simulink model "progetto_condizionatore_pid"  (R2022a)
settings: Solver=VariableStepAuto  StartTime=0.0  StopTime=50000  RelTol=1e-3
values from neighbouring files (symbols this model uses):
  A = [(-gamma_cs/C_c) (gamma_cs/C_c); (gamma_cs/C_s) -((gamma_cs/C_s)+(gamma_sa/C_s))]    [Progetto_condizionatore.m]
  B = [1/C_c; 0]    [Progetto_condizionatore.m]
  C = [0 1]    [Progetto_condizionatore.m]
  C_s = 45225    [Progetto_condizionatore.m]
  D = 0    [Progetto_condizionatore.m]
  gamma_sa = 2.3    [Progetto_condizionatore.m]
  temp_amb = 30    [Progetto_condizionatore.m]
libraries: slpidlib x1
settings Model: Creator=Mattia  LastModifiedBy=Mattia

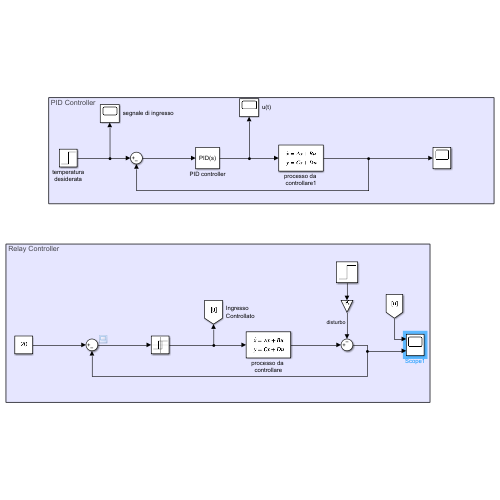
[thumbnail: Simulink's stored preview of the top-level diagram]
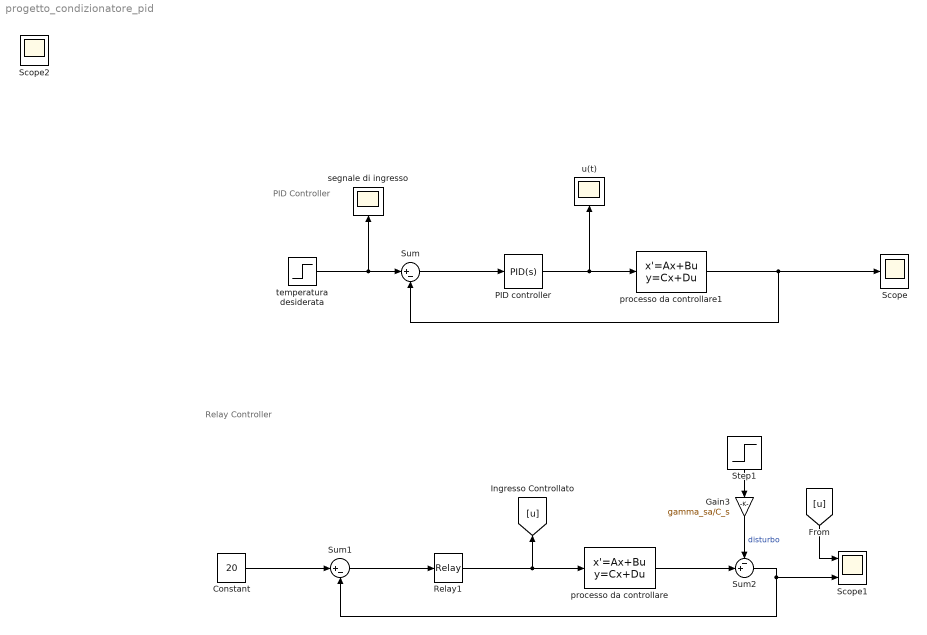
== system progetto_condizionatore_pid ==
  note: Relay Controller
  note: PID Controller
  Constant : Constant  Value=20
  Gain3 : Gain  Gain=gamma_sa/C_s
  PID controller : slpidlib/PID Controller  Controller=PID  Form=Parallel  TimeDomain=Continuous-time  UseExternalTs=off  SampleTime=-1  IntegratorMethod=Forward Euler  FilterMethod=Forward Euler  ControllerParametersSource=internal  P=18  I=0.01  UseKiTs=off  D=0.1  N=100  UseFilter=on  TunerSelectOption=Transfer Function Based (PID Tuner App)  InitialConditionSource=internal  InitialConditionForIntegrator=0  InitialConditionForFilter=0  DifferentiatorICPrevScaledInput=0  ExternalReset=none  TrackingMode=off  Kt=1  LimitOutput=off  SatLimitsSource=internal  UpperSaturationLimit=inf  LowerSaturationLimit=-inf  LinearizeAsGain=on  AntiWindupMode=none  Kb=1  POutMin=[]  POutMax=[]  IOutMin=[]  IOutMax=[]  DOutMin=[]  DOutMax=[]  NOutMin=[]  NOutMax=[]  SumOutMin=[]  SumOutMax=[]  SaturationOutMin=[]  SaturationOutMax=[]  PParamMin=[]  PParamMax=[]  IParamMin=[]  IParamMax=[]  DParamMin=[]  DParamMax=[]  NParamMin=[]  NParamMax=[]  KbParamMin=[]  KbParamMax=[]  KtParamMin=[]  KtParamMax=[]  KbOutMin=[]  KbOutMax=[]  KtOutMin=[]  KtOutMax=[]  IntegratorOutMin=[]  IntegratorOutMax=[]  FilterOutMin=[]  FilterOutMax=[]  SumI1OutMin=[]  SumI1OutMax=[]  SumI2OutMin=[]  SumI2OutMax=[]  SumI3OutMin=[]  SumI3OutMax=[]  SumI4OutMin=[]  SumI4OutMax=[]  SumDOutMin=[]  SumDOutMax=[]  DifferentiatorOutMin=[]  DifferentiatorOutMax=[]  FilterDiffOutCoefMin=[]  FilterDiffOutCoefMax=[]  ReciprocalOutMin=[]  ReciprocalOutMax=[]  SumDenOutMin=[]  SumDenOutMax=[]  SumNumOutMin=[]  SumNumOutMax=[]  DivideOutMin=[]  DivideOutMax=[]  UdiffTsProdOutMin=[]  UdiffTsProdOutMax=[]  NTsProdOutMin=[]  NTsProdOutMax=[]  UintegralTsProdOutMin=[]  UintegralTsProdOutMax=[]  UngainTsProdOutMin=[]  UngainTsProdOutMax=[]  IntegratorContinuousStateAttributes=''  IntegratorStateMustResolveToSignalObject=off  IntegratorRTWStateStorageClass=Auto  FilterContinuousStateAttributes=''  FilterStateMustResolveToSignalObject=off  FilterRTWStateStorageClass=Auto  ParallelPVariant=InternalParameters  IdealPVariant=Disabled  IVariant=InternalParameters  DVariant=InternalParameters  IntegratorVariant=Continuous  SatVariant=Disabled  AWVariant=Passthrough  PCopyVariant=Disabled  TRVariant=Disabled  FdbkBlocksVariant=Forward  IdealPFdbkVariant=Disabled  SatFdbkVariant=Disabled  DerivativeFilterVariant=ContFilter  NVariant=InternalParameters  NCopyVariant=Disabled  FilterICVariant=InternalICsFilter  IntegratorICVariant=InternalICs  ExternalResetVariant=Disabled  TRSumVariant=Passthrough  SumFdbkVariant=Disabled  SumVariant=Sum_PID  TsampFilterVariant=InternalTs  TsampNgainVariant=Passthrough  TsampIntegralVariant=Passthrough  ExternalSaturationOutDataTypeStr=Inherit: Same as second input  aMode=0
  Relay1 : Relay  OnSwitchValue=1  OffSwitchValue=-1  OnOutputValue=55
  Scope : Scope
  Scope1 : Scope  NumInputPorts=2
  Step1 : Step  Time=0  After=temp_amb  SampleTime=0
  Sum : Sum  Inputs=|+-
  Sum1 : Sum  Inputs=|+-
  Sum2 : Sum  Inputs=-+|
  processo da controllare : StateSpace  A=A  B=B  C=C  D=D  InitialCondition=30
  processo da controllare1 : StateSpace  A=A  B=B  C=C  D=D  InitialCondition=30
  segnale di ingresso : Scope
  temperatura desiderata : Step  Time=0  After=20  SampleTime=0
  u(t) : Scope
  Scope2 : Scope
  wires:
  Sum/1 -> PID controller/1
  temperatura desiderata/1 -> segnale di ingresso/1, Sum/1
  processo da controllare1/1 -> Sum/2, Scope/1
  PID controller/1 -> processo da controllare1/1, u(t)/1
  Step1/1 -> Gain3/1
  Gain3/1 -> Sum2/1  "disturbo"
  Sum1/1 -> Relay1/1
  Relay1/1 -> [u], processo da controllare/1
  Constant/1 -> Sum1/1
  processo da controllare/1 -> Sum2/2
  Sum2/1 -> Sum1/2, Scope1/2
  [u] -> Scope1/1
